simulink model "PhysicalLeanBroth"  (R2026a)
settings: Solver=VariableStepAuto
settings Model: DataDictionary=PhysicalInterfaces.sldd  Creator=sarah  LastModifiedBy=sarah

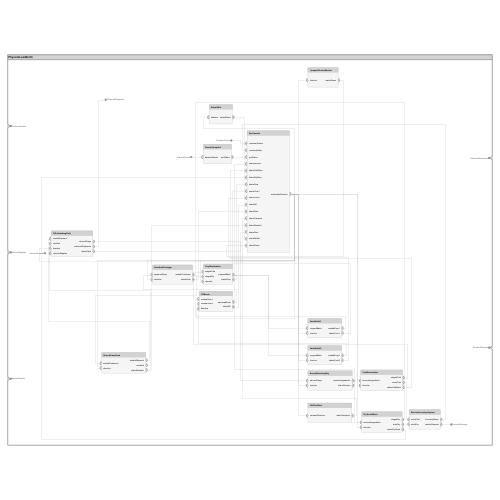
[thumbnail: Simulink's stored preview of the top-level diagram]
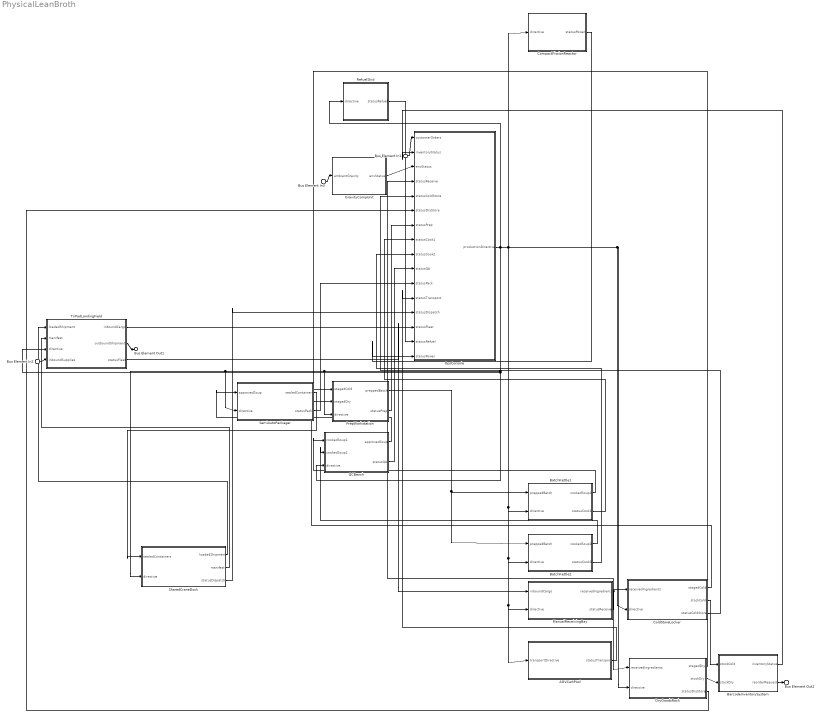
== system PhysicalLeanBroth ==
  Bus Element In1 : Inport  PortName=CustomerOrders
  Bus Element In2 : Inport  Port=2  PortName=InboundSupplies
  Bus Element In3 : Inport  Port=3  PortName=AmbientGravity
  AGVCartPool : Subsystem
      settings: PortSchema="{\"entries\":[{\"content\":{\"headerSize\":26,\"margin\":15,\"minimumSpacing\":25,\"sides\":[{\"content\":{\"connectorIds\":[\"In1\"]},\"type\":\"ConnectorPlacement.EquallySpacedRectSide\",\"uuid\":\"f830f98a-8e8b-4468-adf4-d6eab644987f\"},{\"content\":{\"connectorIds\":[\"Out1\"],\"side\":\"RIGHT\"},\"type\":\"ConnectorPlacement.EquallySpacedRectSide\",\"uuid\":\"7e0d0116-b3ba-4668-b638-30d0f54ba087\"},{\"content\":{\"side\":\"TOP\"},\"type\":\"ConnectorPlacement.EquallySpacedRectSide\",\"uuid\":\"7b4146d3-46d2-45ca-8c34-b106f0d8cedd\"}]},\"type\":\"ConnectorPlacement.EquallySpacedConnector\",\"uuid\":\"3d911b2d-a78f-42ea-b869-5e09982d9f54\"}],\"packageUris\":[\"http://schema.mathworks.com/mf0/Connector/R2020b\"],\"version\":\"1.0\"}"
  BarcodeInventorySystem : Subsystem
      settings: PortSchema="{\"entries\":[{\"content\":{\"headerSize\":26,\"margin\":15,\"minimumSpacing\":25,\"sides\":[{\"content\":{\"connectorIds\":[\"In1\",\"In2\"]},\"type\":\"ConnectorPlacement.EquallySpacedRectSide\",\"uuid\":\"f830f98a-8e8b-4468-adf4-d6eab644987f\"},{\"content\":{\"connectorIds\":[\"Out1\",\"Out2\"],\"side\":\"RIGHT\"},\"type\":\"ConnectorPlacement.EquallySpacedRectSide\",\"uuid\":\"7e0d0116-b3ba-4668-b638-30d0f54ba087\"},{\"content\":{\"side\":\"TOP\"},\"type\":\"ConnectorPlacement.EquallySpacedRectSide\",\"uuid\":\"7b4146d3-46d2-45ca-8c34-b106f0d8cedd\"}]},\"type\":\"ConnectorPlacement.EquallySpacedConnector\",\"uuid\":\"3d911b2d-a78f-42ea-b869-5e09982d9f54\"}],\"packageUris\":[\"http://schema.mathworks.com/mf0/Connector/R2020b\"],\"version\":\"1.0\"}"
  BatchKettle1 : Subsystem
      settings: PortSchema="{\"entries\":[{\"content\":{\"headerSize\":26,\"margin\":15,\"minimumSpacing\":25,\"sides\":[{\"content\":{\"connectorIds\":[\"In1\",\"In2\"]},\"type\":\"ConnectorPlacement.EquallySpacedRectSide\",\"uuid\":\"f830f98a-8e8b-4468-adf4-d6eab644987f\"},{\"content\":{\"connectorIds\":[\"Out1\",\"Out2\"],\"side\":\"RIGHT\"},\"type\":\"ConnectorPlacement.EquallySpacedRectSide\",\"uuid\":\"7e0d0116-b3ba-4668-b638-30d0f54ba087\"},{\"content\":{\"side\":\"TOP\"},\"type\":\"ConnectorPlacement.EquallySpacedRectSide\",\"uuid\":\"7b4146d3-46d2-45ca-8c34-b106f0d8cedd\"}]},\"type\":\"ConnectorPlacement.EquallySpacedConnector\",\"uuid\":\"3d911b2d-a78f-42ea-b869-5e09982d9f54\"}],\"packageUris\":[\"http://schema.mathworks.com/mf0/Connector/R2020b\"],\"version\":\"1.0\"}"
  BatchKettle2 : Subsystem
      settings: PortSchema="{\"entries\":[{\"content\":{\"headerSize\":26,\"margin\":15,\"minimumSpacing\":25,\"sides\":[{\"content\":{\"connectorIds\":[\"In1\",\"In2\"]},\"type\":\"ConnectorPlacement.EquallySpacedRectSide\",\"uuid\":\"f830f98a-8e8b-4468-adf4-d6eab644987f\"},{\"content\":{\"connectorIds\":[\"Out1\",\"Out2\"],\"side\":\"RIGHT\"},\"type\":\"ConnectorPlacement.EquallySpacedRectSide\",\"uuid\":\"7e0d0116-b3ba-4668-b638-30d0f54ba087\"},{\"content\":{\"side\":\"TOP\"},\"type\":\"ConnectorPlacement.EquallySpacedRectSide\",\"uuid\":\"7b4146d3-46d2-45ca-8c34-b106f0d8cedd\"}]},\"type\":\"ConnectorPlacement.EquallySpacedConnector\",\"uuid\":\"3d911b2d-a78f-42ea-b869-5e09982d9f54\"}],\"packageUris\":[\"http://schema.mathworks.com/mf0/Connector/R2020b\"],\"version\":\"1.0\"}"
  ColdStoreLocker : Subsystem
      settings: PortSchema="{\"entries\":[{\"content\":{\"headerSize\":26,\"margin\":15,\"minimumSpacing\":25,\"sides\":[{\"content\":{\"connectorIds\":[\"In1\",\"In2\"]},\"type\":\"ConnectorPlacement.EquallySpacedRectSide\",\"uuid\":\"f830f98a-8e8b-4468-adf4-d6eab644987f\"},{\"content\":{\"connectorIds\":[\"Out1\",\"Out2\",\"Out3\"],\"side\":\"RIGHT\"},\"type\":\"ConnectorPlacement.EquallySpacedRectSide\",\"uuid\":\"7e0d0116-b3ba-4668-b638-30d0f54ba087\"},{\"content\":{\"side\":\"TOP\"},\"type\":\"ConnectorPlacement.EquallySpacedRectSide\",\"uuid\":\"7b4146d3-46d2-45ca-8c34-b106f0d8cedd\"}]},\"type\":\"ConnectorPlacement.EquallySpacedConnector\",\"uuid\":\"3d911b2d-a78f-42ea-b869-5e09982d9f54\"}],\"packageUris\":[\"http://schema.mathworks.com/mf0/Connector/R2020b\"],\"version\":\"1.0\"}"
  CompactFissionReactor : Subsystem
      settings: PortSchema="{\"entries\":[{\"content\":{\"headerSize\":26,\"margin\":15,\"minimumSpacing\":25,\"sides\":[{\"content\":{\"connectorIds\":[\"In1\"]},\"type\":\"ConnectorPlacement.EquallySpacedRectSide\",\"uuid\":\"f830f98a-8e8b-4468-adf4-d6eab644987f\"},{\"content\":{\"connectorIds\":[\"Out1\"],\"side\":\"RIGHT\"},\"type\":\"ConnectorPlacement.EquallySpacedRectSide\",\"uuid\":\"7e0d0116-b3ba-4668-b638-30d0f54ba087\"},{\"content\":{\"side\":\"TOP\"},\"type\":\"ConnectorPlacement.EquallySpacedRectSide\",\"uuid\":\"7b4146d3-46d2-45ca-8c34-b106f0d8cedd\"}]},\"type\":\"ConnectorPlacement.EquallySpacedConnector\",\"uuid\":\"3d911b2d-a78f-42ea-b869-5e09982d9f54\"}],\"packageUris\":[\"http://schema.mathworks.com/mf0/Connector/R2020b\"],\"version\":\"1.0\"}"
  DryGoodsRack : Subsystem
      settings: PortSchema="{\"entries\":[{\"content\":{\"headerSize\":26,\"margin\":15,\"minimumSpacing\":25,\"sides\":[{\"content\":{\"connectorIds\":[\"In1\",\"In2\"]},\"type\":\"ConnectorPlacement.EquallySpacedRectSide\",\"uuid\":\"f830f98a-8e8b-4468-adf4-d6eab644987f\"},{\"content\":{\"connectorIds\":[\"Out1\",\"Out2\",\"Out3\"],\"side\":\"RIGHT\"},\"type\":\"ConnectorPlacement.EquallySpacedRectSide\",\"uuid\":\"7e0d0116-b3ba-4668-b638-30d0f54ba087\"},{\"content\":{\"side\":\"TOP\"},\"type\":\"ConnectorPlacement.EquallySpacedRectSide\",\"uuid\":\"7b4146d3-46d2-45ca-8c34-b106f0d8cedd\"}]},\"type\":\"ConnectorPlacement.EquallySpacedConnector\",\"uuid\":\"3d911b2d-a78f-42ea-b869-5e09982d9f54\"}],\"packageUris\":[\"http://schema.mathworks.com/mf0/Connector/R2020b\"],\"version\":\"1.0\"}"
  GravityCompUnit : Subsystem
      settings: PortSchema="{\"entries\":[{\"content\":{\"headerSize\":26,\"margin\":15,\"minimumSpacing\":25,\"sides\":[{\"content\":{\"connectorIds\":[\"In1\"]},\"type\":\"ConnectorPlacement.EquallySpacedRectSide\",\"uuid\":\"f830f98a-8e8b-4468-adf4-d6eab644987f\"},{\"content\":{\"connectorIds\":[\"Out1\"],\"side\":\"RIGHT\"},\"type\":\"ConnectorPlacement.EquallySpacedRectSide\",\"uuid\":\"7e0d0116-b3ba-4668-b638-30d0f54ba087\"},{\"content\":{\"side\":\"TOP\"},\"type\":\"ConnectorPlacement.EquallySpacedRectSide\",\"uuid\":\"7b4146d3-46d2-45ca-8c34-b106f0d8cedd\"}]},\"type\":\"ConnectorPlacement.EquallySpacedConnector\",\"uuid\":\"3d911b2d-a78f-42ea-b869-5e09982d9f54\"}],\"packageUris\":[\"http://schema.mathworks.com/mf0/Connector/R2020b\"],\"version\":\"1.0\"}"
  ManualReceivingBay : Subsystem
      settings: PortSchema="{\"entries\":[{\"content\":{\"headerSize\":26,\"margin\":15,\"minimumSpacing\":25,\"sides\":[{\"content\":{\"connectorIds\":[\"In1\",\"In2\"]},\"type\":\"ConnectorPlacement.EquallySpacedRectSide\",\"uuid\":\"f830f98a-8e8b-4468-adf4-d6eab644987f\"},{\"content\":{\"connectorIds\":[\"Out1\",\"Out2\"],\"side\":\"RIGHT\"},\"type\":\"ConnectorPlacement.EquallySpacedRectSide\",\"uuid\":\"7e0d0116-b3ba-4668-b638-30d0f54ba087\"},{\"content\":{\"side\":\"TOP\"},\"type\":\"ConnectorPlacement.EquallySpacedRectSide\",\"uuid\":\"7b4146d3-46d2-45ca-8c34-b106f0d8cedd\"}]},\"type\":\"ConnectorPlacement.EquallySpacedConnector\",\"uuid\":\"3d911b2d-a78f-42ea-b869-5e09982d9f54\"}],\"packageUris\":[\"http://schema.mathworks.com/mf0/Connector/R2020b\"],\"version\":\"1.0\"}"
  OpsConsole : Subsystem
      settings: PortSchema="{\"entries\":[{\"content\":{\"headerSize\":26,\"margin\":15,\"minimumSpacing\":25,\"sides\":[{\"content\":{\"connectorIds\":[\"In1\",\"In2\",\"In3\",\"In4\",\"In5\",\"In6\",\"In7\",\"In8\",\"In9\",\"In10\",\"In11\",\"In12\",\"In13\",\"In14\",\"In15\",\"In16\"]},\"type\":\"ConnectorPlacement.EquallySpacedRectSide\",\"uuid\":\"f830f98a-8e8b-4468-adf4-d6eab644987f\"},{\"content\":{\"connectorIds\":[\"Out1\"],\"side\":\"RIGHT\"},\"type\":\"ConnectorPlacement.EquallySpacedRectSide\",\"uuid\":\"7e0d0116-b3ba-4668-b638-30d0f54ba087\"},{\"content\":{\"side\":\"TOP\"},\"type\":\"ConnectorPlacement.EquallySpacedRectSide\",\"uuid\":\"7b4146d3-46d2-45ca-8c34-b106f0d8cedd\"}]},\"type\":\"ConnectorPlacement.EquallySpacedConnector\",\"uuid\":\"3d911b2d-a78f-42ea-b869-5e09982d9f54\"}],\"packageUris\":[\"http://schema.mathworks.com/mf0/Connector/R2020b\"],\"version\":\"1.0\"}"
  PrepWorkstation : Subsystem
      settings: PortSchema="{\"entries\":[{\"content\":{\"headerSize\":26,\"margin\":15,\"minimumSpacing\":25,\"sides\":[{\"content\":{\"connectorIds\":[\"In1\",\"In2\",\"In3\"]},\"type\":\"ConnectorPlacement.EquallySpacedRectSide\",\"uuid\":\"f830f98a-8e8b-4468-adf4-d6eab644987f\"},{\"content\":{\"connectorIds\":[\"Out1\",\"Out2\"],\"side\":\"RIGHT\"},\"type\":\"ConnectorPlacement.EquallySpacedRectSide\",\"uuid\":\"7e0d0116-b3ba-4668-b638-30d0f54ba087\"},{\"content\":{\"side\":\"TOP\"},\"type\":\"ConnectorPlacement.EquallySpacedRectSide\",\"uuid\":\"7b4146d3-46d2-45ca-8c34-b106f0d8cedd\"}]},\"type\":\"ConnectorPlacement.EquallySpacedConnector\",\"uuid\":\"3d911b2d-a78f-42ea-b869-5e09982d9f54\"}],\"packageUris\":[\"http://schema.mathworks.com/mf0/Connector/R2020b\"],\"version\":\"1.0\"}"
  QCBench : Subsystem
      settings: PortSchema="{\"entries\":[{\"content\":{\"headerSize\":26,\"margin\":15,\"minimumSpacing\":25,\"sides\":[{\"content\":{\"connectorIds\":[\"In1\",\"In2\",\"In3\"]},\"type\":\"ConnectorPlacement.EquallySpacedRectSide\",\"uuid\":\"f830f98a-8e8b-4468-adf4-d6eab644987f\"},{\"content\":{\"connectorIds\":[\"Out1\",\"Out2\"],\"side\":\"RIGHT\"},\"type\":\"ConnectorPlacement.EquallySpacedRectSide\",\"uuid\":\"7e0d0116-b3ba-4668-b638-30d0f54ba087\"},{\"content\":{\"side\":\"TOP\"},\"type\":\"ConnectorPlacement.EquallySpacedRectSide\",\"uuid\":\"7b4146d3-46d2-45ca-8c34-b106f0d8cedd\"}]},\"type\":\"ConnectorPlacement.EquallySpacedConnector\",\"uuid\":\"3d911b2d-a78f-42ea-b869-5e09982d9f54\"}],\"packageUris\":[\"http://schema.mathworks.com/mf0/Connector/R2020b\"],\"version\":\"1.0\"}"
  RefuelSkid : Subsystem
      settings: PortSchema="{\"entries\":[{\"content\":{\"headerSize\":26,\"margin\":15,\"minimumSpacing\":25,\"sides\":[{\"content\":{\"connectorIds\":[\"In1\"]},\"type\":\"ConnectorPlacement.EquallySpacedRectSide\",\"uuid\":\"f830f98a-8e8b-4468-adf4-d6eab644987f\"},{\"content\":{\"connectorIds\":[\"Out1\"],\"side\":\"RIGHT\"},\"type\":\"ConnectorPlacement.EquallySpacedRectSide\",\"uuid\":\"7e0d0116-b3ba-4668-b638-30d0f54ba087\"},{\"content\":{\"side\":\"TOP\"},\"type\":\"ConnectorPlacement.EquallySpacedRectSide\",\"uuid\":\"7b4146d3-46d2-45ca-8c34-b106f0d8cedd\"}]},\"type\":\"ConnectorPlacement.EquallySpacedConnector\",\"uuid\":\"3d911b2d-a78f-42ea-b869-5e09982d9f54\"}],\"packageUris\":[\"http://schema.mathworks.com/mf0/Connector/R2020b\"],\"version\":\"1.0\"}"
  SemiAutoPackager : Subsystem
      settings: PortSchema="{\"entries\":[{\"content\":{\"headerSize\":26,\"margin\":15,\"minimumSpacing\":25,\"sides\":[{\"content\":{\"connectorIds\":[\"In1\",\"In2\"]},\"type\":\"ConnectorPlacement.EquallySpacedRectSide\",\"uuid\":\"f830f98a-8e8b-4468-adf4-d6eab644987f\"},{\"content\":{\"connectorIds\":[\"Out1\",\"Out2\"],\"side\":\"RIGHT\"},\"type\":\"ConnectorPlacement.EquallySpacedRectSide\",\"uuid\":\"7e0d0116-b3ba-4668-b638-30d0f54ba087\"},{\"content\":{\"side\":\"TOP\"},\"type\":\"ConnectorPlacement.EquallySpacedRectSide\",\"uuid\":\"7b4146d3-46d2-45ca-8c34-b106f0d8cedd\"}]},\"type\":\"ConnectorPlacement.EquallySpacedConnector\",\"uuid\":\"3d911b2d-a78f-42ea-b869-5e09982d9f54\"}],\"packageUris\":[\"http://schema.mathworks.com/mf0/Connector/R2020b\"],\"version\":\"1.0\"}"
  SharedCraneDock : Subsystem
      settings: PortSchema="{\"entries\":[{\"content\":{\"headerSize\":26,\"margin\":15,\"minimumSpacing\":25,\"sides\":[{\"content\":{\"connectorIds\":[\"In1\",\"In2\"]},\"type\":\"ConnectorPlacement.EquallySpacedRectSide\",\"uuid\":\"f830f98a-8e8b-4468-adf4-d6eab644987f\"},{\"content\":{\"connectorIds\":[\"Out1\",\"Out2\",\"Out3\"],\"side\":\"RIGHT\"},\"type\":\"ConnectorPlacement.EquallySpacedRectSide\",\"uuid\":\"7e0d0116-b3ba-4668-b638-30d0f54ba087\"},{\"content\":{\"side\":\"TOP\"},\"type\":\"ConnectorPlacement.EquallySpacedRectSide\",\"uuid\":\"7b4146d3-46d2-45ca-8c34-b106f0d8cedd\"}]},\"type\":\"ConnectorPlacement.EquallySpacedConnector\",\"uuid\":\"3d911b2d-a78f-42ea-b869-5e09982d9f54\"}],\"packageUris\":[\"http://schema.mathworks.com/mf0/Connector/R2020b\"],\"version\":\"1.0\"}"
  TriPadLandingField : Subsystem
      settings: PortSchema="{\"entries\":[{\"content\":{\"headerSize\":26,\"margin\":15,\"minimumSpacing\":25,\"sides\":[{\"content\":{\"connectorIds\":[\"In1\",\"In2\",\"In3\",\"In4\"]},\"type\":\"ConnectorPlacement.EquallySpacedRectSide\",\"uuid\":\"f830f98a-8e8b-4468-adf4-d6eab644987f\"},{\"content\":{\"connectorIds\":[\"Out1\",\"Out2\",\"Out3\"],\"side\":\"RIGHT\"},\"type\":\"ConnectorPlacement.EquallySpacedRectSide\",\"uuid\":\"7e0d0116-b3ba-4668-b638-30d0f54ba087\"},{\"content\":{\"side\":\"TOP\"},\"type\":\"ConnectorPlacement.EquallySpacedRectSide\",\"uuid\":\"7b4146d3-46d2-45ca-8c34-b106f0d8cedd\"}]},\"type\":\"ConnectorPlacement.EquallySpacedConnector\",\"uuid\":\"3d911b2d-a78f-42ea-b869-5e09982d9f54\"}],\"packageUris\":[\"http://schema.mathworks.com/mf0/Connector/R2020b\"],\"version\":\"1.0\"}"
  Bus Element Out1 : Outport  PortName=OutboundShipments
  Bus Element Out2 : Outport  Port=2  PortName=ReorderRequests
  wires:
  TriPadLandingField/2(outboundShipments) -> Bus Element Out1/1
  Bus Element In2/1 -> TriPadLandingField/4(inboundSupplies)
  SharedCraneDock/3(statusDispatch) -> OpsConsole/13(statusDispatch)
  TriPadLandingField/1(inboundCargo) -> ManualReceivingBay/1(inboundCargo)
  TriPadLandingField/3(statusFleet) -> OpsConsole/14(statusFleet)
  SharedCraneDock/1(loadedShipment) -> TriPadLandingField/1(loadedShipment)
  Bus Element In3/1 -> GravityCompUnit/1(ambientGravity)
  SharedCraneDock/2(manifest) -> TriPadLandingField/2(manifest)
  SemiAutoPackager/1(sealedContainers) -> SharedCraneDock/1(sealedContainers)
  SemiAutoPackager/2(statusPack) -> OpsConsole/11(statusPack)
  RefuelSkid/1(statusRefuel) -> OpsConsole/15(statusRefuel)
  Bus Element In1/1 -> OpsConsole/1(customerOrders)
  GravityCompUnit/1(envStatus) -> OpsConsole/3(envStatus)
  PrepWorkstation/1(preppedBatch) -> BatchKettle2/1(preppedBatch), BatchKettle1/1(preppedBatch)
  ManualReceivingBay/1(receivedIngredients) -> ColdStoreLocker/1(receivedIngredients), DryGoodsRack/1(receivedIngredients)
  PrepWorkstation/2(statusPrep) -> OpsConsole/7(statusPrep)
  QCBench/1(approvedSoup) -> SemiAutoPackager/1(approvedSoup)
  QCBench/2(statusQA) -> OpsConsole/10(statusQA)
  BarcodeInventorySystem/1(inventoryStatus) -> OpsConsole/2(inventoryStatus)
  OpsConsole/1(productionDirective) -> QCBench/3(directive), TriPadLandingField/3(directive), SharedCraneDock/2(directive), SemiAutoPackager/2(directive), PrepWorkstation/3(directive), ManualReceivingBay/2(directive), AGVCartPool/1(transportDirective), BatchKettle2/2(directive), BatchKettle1/2(directive), ColdStoreLocker/2(directive), DryGoodsRack/2(directive), CompactFissionReactor/1(directive), RefuelSkid/1(directive)
  CompactFissionReactor/1(statusPower) -> OpsConsole/16(statusPower)
  BatchKettle1/1(cookedSoup1) -> QCBench/1(cookedSoup1)
  ColdStoreLocker/1(stagedCold) -> PrepWorkstation/1(stagedCold)
  BatchKettle1/2(statusCook1) -> OpsConsole/8(statusCook1)
  BatchKettle2/1(cookedSoup2) -> QCBench/2(cookedSoup2)
  BatchKettle2/2(statusCook2) -> OpsConsole/9(statusCook2)
  ManualReceivingBay/2(statusReceive) -> OpsConsole/4(statusReceive)
  AGVCartPool/1(statusTransport) -> OpsConsole/12(statusTransport)
  ColdStoreLocker/2(stockCold) -> BarcodeInventorySystem/1(stockCold)
  ColdStoreLocker/3(statusColdStore) -> OpsConsole/5(statusColdStore)
  DryGoodsRack/1(stagedDry) -> PrepWorkstation/2(stagedDry)
  DryGoodsRack/2(stockDry) -> BarcodeInventorySystem/2(stockDry)
  DryGoodsRack/3(statusDryStore) -> OpsConsole/6(statusDryStore)
  BarcodeInventorySystem/2(reorderRequest) -> Bus Element Out2/1

== system PhysicalLeanBroth/AGVCartPool ==
  Bus Element In1 : Inport  PortName=transportDirective
  Bus Element Out1 : Outport  PortName=statusTransport

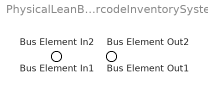
== system PhysicalLeanBroth/BarcodeInventorySystem ==
  Bus Element In1 : Inport  PortName=stockCold
  Bus Element In2 : Inport  Port=2  PortName=stockDry
  Bus Element Out1 : Outport  PortName=inventoryStatus
  Bus Element Out2 : Outport  Port=2  PortName=reorderRequest

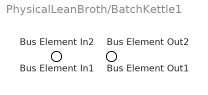
== system PhysicalLeanBroth/BatchKettle1 ==
  Bus Element In1 : Inport  PortName=preppedBatch
  Bus Element In2 : Inport  Port=2  PortName=directive
  Bus Element Out1 : Outport  PortName=cookedSoup1
  Bus Element Out2 : Outport  Port=2  PortName=statusCook1

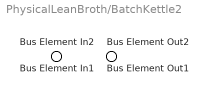
== system PhysicalLeanBroth/BatchKettle2 ==
  Bus Element In1 : Inport  PortName=preppedBatch
  Bus Element In2 : Inport  Port=2  PortName=directive
  Bus Element Out1 : Outport  PortName=cookedSoup2
  Bus Element Out2 : Outport  Port=2  PortName=statusCook2

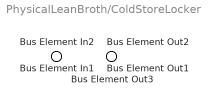
== system PhysicalLeanBroth/ColdStoreLocker ==
  Bus Element In1 : Inport  PortName=receivedIngredients
  Bus Element In2 : Inport  Port=2  PortName=directive
  Bus Element Out1 : Outport  PortName=stagedCold
  Bus Element Out2 : Outport  Port=2  PortName=stockCold
  Bus Element Out3 : Outport  Port=3  PortName=statusColdStore

== system PhysicalLeanBroth/CompactFissionReactor ==
  Bus Element In1 : Inport  PortName=directive
  Bus Element Out1 : Outport  PortName=statusPower

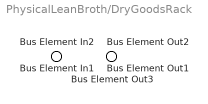
== system PhysicalLeanBroth/DryGoodsRack ==
  Bus Element In1 : Inport  PortName=receivedIngredients
  Bus Element In2 : Inport  Port=2  PortName=directive
  Bus Element Out1 : Outport  PortName=stagedDry
  Bus Element Out2 : Outport  Port=2  PortName=stockDry
  Bus Element Out3 : Outport  Port=3  PortName=statusDryStore

== system PhysicalLeanBroth/GravityCompUnit ==
  Bus Element In1 : Inport  PortName=ambientGravity
  Bus Element Out1 : Outport  PortName=envStatus

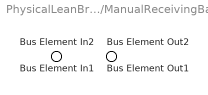
== system PhysicalLeanBroth/ManualReceivingBay ==
  Bus Element In1 : Inport  PortName=inboundCargo
  Bus Element In2 : Inport  Port=2  PortName=directive
  Bus Element Out1 : Outport  PortName=receivedIngredients
  Bus Element Out2 : Outport  Port=2  PortName=statusReceive

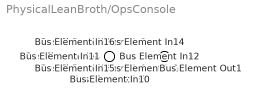
== system PhysicalLeanBroth/OpsConsole ==
  Bus Element In1 : Inport  PortName=customerOrders
  Bus Element In2 : Inport  Port=2  PortName=inventoryStatus
  Bus Element In3 : Inport  Port=3  PortName=envStatus
  Bus Element In4 : Inport  Port=4  PortName=statusReceive
  Bus Element In5 : Inport  Port=5  PortName=statusColdStore
  Bus Element In6 : Inport  Port=6  PortName=statusDryStore
  Bus Element In7 : Inport  Port=7  PortName=statusPrep
  Bus Element In8 : Inport  Port=8  PortName=statusCook1
  Bus Element In9 : Inport  Port=9  PortName=statusCook2
  Bus Element In10 : Inport  Port=10  PortName=statusQA
  Bus Element In11 : Inport  Port=11  PortName=statusPack
  Bus Element In12 : Inport  Port=12  PortName=statusTransport
  Bus Element In13 : Inport  Port=13  PortName=statusDispatch
  Bus Element In14 : Inport  Port=14  PortName=statusFleet
  Bus Element In15 : Inport  Port=15  PortName=statusRefuel
  Bus Element In16 : Inport  Port=16  PortName=statusPower
  Bus Element Out1 : Outport  PortName=productionDirective

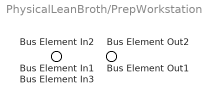
== system PhysicalLeanBroth/PrepWorkstation ==
  Bus Element In1 : Inport  PortName=stagedCold
  Bus Element In2 : Inport  Port=2  PortName=stagedDry
  Bus Element In3 : Inport  Port=3  PortName=directive
  Bus Element Out1 : Outport  PortName=preppedBatch
  Bus Element Out2 : Outport  Port=2  PortName=statusPrep

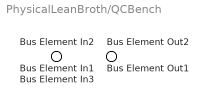
== system PhysicalLeanBroth/QCBench ==
  Bus Element In1 : Inport  PortName=cookedSoup1
  Bus Element In2 : Inport  Port=2  PortName=cookedSoup2
  Bus Element In3 : Inport  Port=3  PortName=directive
  Bus Element Out1 : Outport  PortName=approvedSoup
  Bus Element Out2 : Outport  Port=2  PortName=statusQA

== system PhysicalLeanBroth/RefuelSkid ==
  Bus Element In1 : Inport  PortName=directive
  Bus Element Out1 : Outport  PortName=statusRefuel

== system PhysicalLeanBroth/SemiAutoPackager ==
  Bus Element In1 : Inport  PortName=approvedSoup
  Bus Element In2 : Inport  Port=2  PortName=directive
  Bus Element Out1 : Outport  PortName=sealedContainers
  Bus Element Out2 : Outport  Port=2  PortName=statusPack

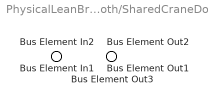
== system PhysicalLeanBroth/SharedCraneDock ==
  Bus Element In1 : Inport  PortName=sealedContainers
  Bus Element In2 : Inport  Port=2  PortName=directive
  Bus Element Out1 : Outport  PortName=loadedShipment
  Bus Element Out2 : Outport  Port=2  PortName=manifest
  Bus Element Out3 : Outport  Port=3  PortName=statusDispatch

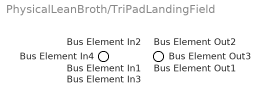
== system PhysicalLeanBroth/TriPadLandingField ==
  Bus Element In1 : Inport  PortName=loadedShipment
  Bus Element In2 : Inport  Port=2  PortName=manifest
  Bus Element In3 : Inport  Port=3  PortName=directive
  Bus Element In4 : Inport  Port=4  PortName=inboundSupplies
  Bus Element Out1 : Outport  PortName=inboundCargo
  Bus Element Out2 : Outport  Port=2  PortName=outboundShipments
  Bus Element Out3 : Outport  Port=3  PortName=statusFleet
